simulink model "controladores_analiseComparacao_PIDTuner_and_projetado"  (R2020a)
settings: Solver=VariableStepAuto  StartTime=0.0  StopTime=10.0  RelTol=1e-3
libraries: simulink x2
settings Model: Creator=estef  LastModifiedBy=crist

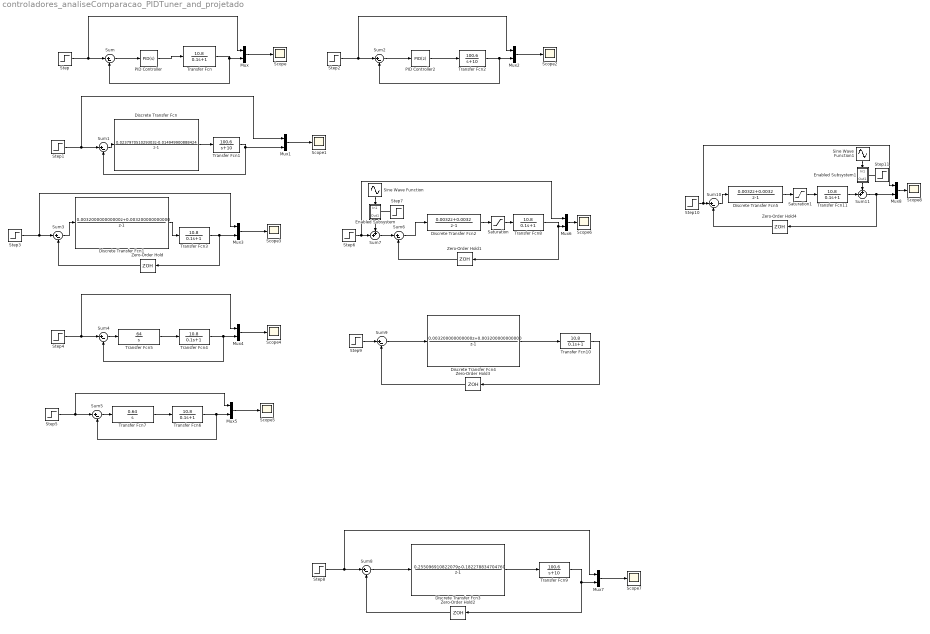
== system controladores_analiseComparacao_PIDTuner_and_projetado ==
  Discrete Transfer Fcn : DiscreteTransferFcn  Numerator=[0.023797051029303 -0.014949900888424]  Denominator=[1 -1]
  Discrete Transfer Fcn1 : DiscreteTransferFcn  Numerator=[0.003200000000000 0.003200000000000]  Denominator=[1 -1]
  Discrete Transfer Fcn2 : DiscreteTransferFcn  Numerator=[0.0032 0.0032]  Denominator=[1 -1]
  Discrete Transfer Fcn3 : DiscreteTransferFcn  Numerator=[0.255096910822079 -0.182278834704760]  Denominator=[1 -1]
  Discrete Transfer Fcn4 : DiscreteTransferFcn  Numerator=[0.003200000000000 0.003200000000000]  Denominator=[1 -1]
  Discrete Transfer Fcn5 : DiscreteTransferFcn  Numerator=[0.0032 0.0032]  Denominator=[1 -1]
  Enabled Subsystem : Subsystem  TreatAsAtomicUnit=on
  Enabled Subsystem1 : Subsystem  TreatAsAtomicUnit=on
  Mux{,1..8} (9 alike) : Mux  Inputs=2
  PID Controller : simulink/Continuous/PID Controller  Controller=PID  Form=Parallel  TimeDomain=Continuous-time  UseExternalTs=off  SampleTime=0.01  IntegratorMethod=Forward Euler  FilterMethod=Forward Euler  ControllerParametersSource=internal  P=0  I=0.64  D=0  UseFilter=on  N=100  TunerSelectOption=Transfer Function Based (PID Tuner App)  InitialConditionSource=internal  InitialConditionForIntegrator=0  InitialConditionForFilter=0  DifferentiatorICPrevScaledInput=0  ExternalReset=none  TrackingMode=off  Kt=1  LimitOutput=off  UpperSaturationLimit=inf  LowerSaturationLimit=-inf  LinearizeAsGain=on  AntiWindupMode=none  Kb=1  POutMin=[]  POutMax=[]  IOutMin=[]  IOutMax=[]  DOutMin=[]  DOutMax=[]  NOutMin=[]  NOutMax=[]  SumOutMin=[]  SumOutMax=[]  SaturationOutMin=[]  SaturationOutMax=[]  PParamMin=[]  PParamMax=[]  IParamMin=[]  IParamMax=[]  DParamMin=[]  DParamMax=[]  NParamMin=[]  NParamMax=[]  KbParamMin=[]  KbParamMax=[]  KtParamMin=[]  KtParamMax=[]  KbOutMin=[]  KbOutMax=[]  KtOutMin=[]  KtOutMax=[]  IntegratorOutMin=[]  IntegratorOutMax=[]  FilterOutMin=[]  FilterOutMax=[]  SumI1OutMin=[]  SumI1OutMax=[]  SumI2OutMin=[]  SumI2OutMax=[]  SumI3OutMin=[]  SumI3OutMax=[]  SumI4OutMin=[]  SumI4OutMax=[]  SumDOutMin=[]  SumDOutMax=[]  DifferentiatorOutMin=[]  DifferentiatorOutMax=[]  FilterDiffOutCoefMin=[]  FilterDiffOutCoefMax=[]  ReciprocalOutMin=[]  ReciprocalOutMax=[]  SumDenOutMin=[]  SumDenOutMax=[]  SumNumOutMin=[]  SumNumOutMax=[]  DivideOutMin=[]  DivideOutMax=[]  UdiffTsProdOutMin=[]  UdiffTsProdOutMax=[]  NTsProdOutMin=[]  NTsProdOutMax=[]  UintegralTsProdOutMin=[]  UintegralTsProdOutMax=[]  UngainTsProdOutMin=[]  UngainTsProdOutMax=[]  IntegratorContinuousStateAttributes=''  IntegratorStateMustResolveToSignalObject=off  IntegratorRTWStateStorageClass=Auto  FilterContinuousStateAttributes=''  FilterStateMustResolveToSignalObject=off  FilterRTWStateStorageClass=Auto  ParallelPVariant=InternalParameters  IdealPVariant=Disabled  IVariant=InternalParameters  DVariant=InternalParameters  IntegratorVariant=Continuous  SatVariant=Disabled  AWVariant=Passthrough  PCopyVariant=Disabled  TRVariant=Disabled  FdbkBlocksVariant=Forward  IdealPFdbkVariant=Disabled  SatFdbkVariant=Disabled  DerivativeFilterVariant=ContFilter  NVariant=InternalParameters  NCopyVariant=Disabled  FilterICVariant=InternalICsFilter  IntegratorICVariant=InternalICs  ExternalResetVariant=Disabled  TRSumVariant=Passthrough  SumFdbkVariant=Disabled  SumVariant=Sum_PID  TsampFilterVariant=InternalTs  TsampNgainVariant=Passthrough  TsampIntegralVariant=Passthrough
  PID Controller2 : simulink/Continuous/PID Controller  Controller=PID  Form=Parallel  TimeDomain=Discrete-time  UseExternalTs=off  SampleTime=-1  IntegratorMethod=Forward Euler  FilterMethod=Forward Euler  ControllerParametersSource=internal  P=1  I=1  D=0  UseFilter=on  N=100  TunerSelectOption=Transfer Function Based (PID Tuner App)  InitialConditionSource=internal  InitialConditionForIntegrator=0  InitialConditionForFilter=0  DifferentiatorICPrevScaledInput=0  ExternalReset=none  TrackingMode=off  Kt=1  LimitOutput=off  UpperSaturationLimit=inf  LowerSaturationLimit=-inf  LinearizeAsGain=on  AntiWindupMode=none  Kb=1  POutMin=[]  POutMax=[]  IOutMin=[]  IOutMax=[]  DOutMin=[]  DOutMax=[]  NOutMin=[]  NOutMax=[]  SumOutMin=[]  SumOutMax=[]  SaturationOutMin=[]  SaturationOutMax=[]  PParamMin=[]  PParamMax=[]  IParamMin=[]  IParamMax=[]  DParamMin=[]  DParamMax=[]  NParamMin=[]  NParamMax=[]  KbParamMin=[]  KbParamMax=[]  KtParamMin=[]  KtParamMax=[]  KbOutMin=[]  KbOutMax=[]  KtOutMin=[]  KtOutMax=[]  IntegratorOutMin=[]  IntegratorOutMax=[]  FilterOutMin=[]  FilterOutMax=[]  SumI1OutMin=[]  SumI1OutMax=[]  SumI2OutMin=[]  SumI2OutMax=[]  SumI3OutMin=[]  SumI3OutMax=[]  SumI4OutMin=[]  SumI4OutMax=[]  SumDOutMin=[]  SumDOutMax=[]  DifferentiatorOutMin=[]  DifferentiatorOutMax=[]  FilterDiffOutCoefMin=[]  FilterDiffOutCoefMax=[]  ReciprocalOutMin=[]  ReciprocalOutMax=[]  SumDenOutMin=[]  SumDenOutMax=[]  SumNumOutMin=[]  SumNumOutMax=[]  DivideOutMin=[]  DivideOutMax=[]  UdiffTsProdOutMin=[]  UdiffTsProdOutMax=[]  NTsProdOutMin=[]  NTsProdOutMax=[]  UintegralTsProdOutMin=[]  UintegralTsProdOutMax=[]  UngainTsProdOutMin=[]  UngainTsProdOutMax=[]  IntegratorContinuousStateAttributes=''  IntegratorStateMustResolveToSignalObject=off  IntegratorRTWStateStorageClass=Auto  FilterContinuousStateAttributes=''  FilterStateMustResolveToSignalObject=off  FilterRTWStateStorageClass=Auto  ParallelPVariant=InternalParameters  IdealPVariant=Disabled  IVariant=InternalParameters  DVariant=InternalParameters  IntegratorVariant=Discrete  SatVariant=Disabled  AWVariant=Passthrough  PCopyVariant=Disabled  TRVariant=Disabled  FdbkBlocksVariant=Forward  IdealPFdbkVariant=Disabled  SatFdbkVariant=Disabled  DerivativeFilterVariant=ForwardEulerFilter  NVariant=InternalParameters  NCopyVariant=Disabled  FilterICVariant=InternalICsFilter  IntegratorICVariant=InternalICs  ExternalResetVariant=Disabled  TRSumVariant=Passthrough  SumFdbkVariant=Disabled  SumVariant=Sum_PID  TsampFilterVariant=InternalTs  TsampNgainVariant=Passthrough  TsampIntegralVariant=Passthrough
  Saturation : Saturate  UpperLimit=1  LowerLimit=0
  Saturation1 : Saturate  UpperLimit=1  LowerLimit=0
  Scope{,1..8} (9 alike) : Scope
  Sine Wave Function : Sin  Amplitude=0.2  Frequency=50  SampleTime=0
  Sine Wave Function1 : Sin  Amplitude=0.2  Frequency=50  SampleTime=0
  Step{,1..11} (12 alike) : Step  SampleTime=0
  Sum{,1..6,8..10} (10 alike) : Sum  Inputs=|+-
  Sum11 : Sum  Inputs=++|
  Sum7 : Sum  Inputs=++|
  Transfer Fcn{,3..4,6,8,10..11} (7 alike) : TransferFcn  Numerator=[10.8]  Denominator=[0.1 1]
  Transfer Fcn1 : TransferFcn  Numerator=[100.6]  Denominator=[1 10]
  Transfer Fcn2 : TransferFcn  Numerator=[100.6]  Denominator=[1 10]
  Transfer Fcn5 : TransferFcn  Numerator=[64]  Denominator=[1 0]
  Transfer Fcn7 : TransferFcn  Numerator=[0.64]  Denominator=[1 0]
  Transfer Fcn9 : TransferFcn  Numerator=[100.6]  Denominator=[1 10]
  Zero-Order Hold{,1,3..4} (4 alike) : ZeroOrderHold  SampleTime=0.01
  Zero-Order Hold2 : ZeroOrderHold  SampleTime=-1
  wires:
  Mux/1 -> Scope/1
  Transfer Fcn/1 -> Sum/2, Mux/2
  PID Controller/1 -> Transfer Fcn/1
  Sum/1 -> PID Controller/1
  Step/1 -> Mux/1, Sum/1
  Sum1/1 -> Discrete Transfer Fcn/1
  Discrete Transfer Fcn/1 -> Transfer Fcn1/1
  Step1/1 -> Mux1/1, Sum1/1
  Transfer Fcn1/1 -> Mux1/2, Sum1/2
  Sum2/1 -> PID Controller2/1
  PID Controller2/1 -> Transfer Fcn2/1
  Step2/1 -> Mux2/1, Sum2/1
  Mux2/1 -> Scope2/1
  Transfer Fcn2/1 -> Sum2/2, Mux2/2
  Mux3/1 -> Scope3/1
  Step3/1 -> Sum3/1, Mux3/1
  Transfer Fcn3/1 -> Zero-Order Hold/1, Mux3/2
  Transfer Fcn4/1 -> Sum4/2, Mux4/2
  Step4/1 -> Mux4/1, Sum4/1
  Mux4/1 -> Scope4/1
  Transfer Fcn5/1 -> Transfer Fcn4/1
  Sum4/1 -> Transfer Fcn5/1
  Mux1/1 -> Scope1/1
  Discrete Transfer Fcn1/1 -> Transfer Fcn3/1
  Sum3/1 -> Discrete Transfer Fcn1/1
  Sum5/1 -> Transfer Fcn7/1
  Transfer Fcn7/1 -> Transfer Fcn6/1
  Mux5/1 -> Scope5/1
  Transfer Fcn6/1 -> Sum5/2, Mux5/2
  Step5/1 -> Mux5/1, Sum5/1
  Zero-Order Hold/1 -> Sum3/2
  Zero-Order Hold1/1 -> Sum6/2
  Sum6/1 -> Discrete Transfer Fcn2/1
  Mux6/1 -> Scope6/1
  Transfer Fcn8/1 -> Mux6/2, Zero-Order Hold1/1
  Sum7/1 -> Sum6/1
  Step6/1 -> Mux6/1, Sum7/2
  Sine Wave Function/1 -> Enabled Subsystem/1(In1)
  Step7/1 -> Enabled Subsystem/Enable
  Enabled Subsystem/1(Out1) -> Sum7/1
  Zero-Order Hold2/1 -> Sum8/2
  Discrete Transfer Fcn3/1 -> Transfer Fcn9/1
  Step8/1 -> Sum8/1, Mux7/1
  Transfer Fcn9/1 -> Zero-Order Hold2/1, Mux7/2
  Mux7/1 -> Scope7/1
  Sum8/1 -> Discrete Transfer Fcn3/1
  Step9/1 -> Sum9/1
  Zero-Order Hold3/1 -> Sum9/2
  Transfer Fcn10/1 -> Zero-Order Hold3/1
  Discrete Transfer Fcn4/1 -> Transfer Fcn10/1
  Sum9/1 -> Discrete Transfer Fcn4/1
  Discrete Transfer Fcn2/1 -> Saturation/1
  Saturation/1 -> Transfer Fcn8/1
  Saturation1/1 -> Transfer Fcn11/1
  Step10/1 -> Sum10/1, Mux8/1
  Zero-Order Hold4/1 -> Sum10/2
  Discrete Transfer Fcn5/1 -> Saturation1/1
  Mux8/1 -> Scope8/1
  Sum10/1 -> Discrete Transfer Fcn5/1
  Enabled Subsystem1/1(Out1) -> Sum11/1
  Step11/1 -> Enabled Subsystem1/Enable
  Sine Wave Function1/1 -> Enabled Subsystem1/1(In1)
  Transfer Fcn11/1 -> Sum11/2
  Sum11/1 -> Zero-Order Hold4/1, Mux8/2

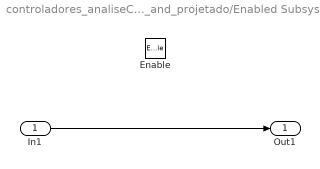
== system controladores_analiseComparacao_PIDTuner_and_projetado/Enabled Subsystem ==
  In1 : Inport
  Enable : EnablePort
  Out1 : Outport
  wires:
  In1/1 -> Out1/1

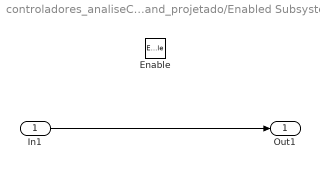
== system controladores_analiseComparacao_PIDTuner_and_projetado/Enabled Subsystem1 ==
  In1 : Inport
  Enable : EnablePort
  Out1 : Outport
  wires:
  In1/1 -> Out1/1
